simulink model "is95fwdchcodec"  (Simulink 4.00)
settings: Solver=VariableStepDiscrete  SolverMode=SingleTasking  StartTime=0.0  StopTime=20.0  RelTol=1e-3  AbsTol=1e-6
undefined symbols (not defined in the file or in its folder): slcm
libraries: cdmalib x8, dspsrcs2 x3, dspmtrx2 x2, commsink x2, commchan x1
settings Model: Creator=rkumar  LastModifiedBy=akansal  SaveTime=off  SaveOutput=off  LimitDataPoints=off  ExtModeTrigMode=oneshot  ExtModeArmWhenConnect=off  BlockReductionOpt=off

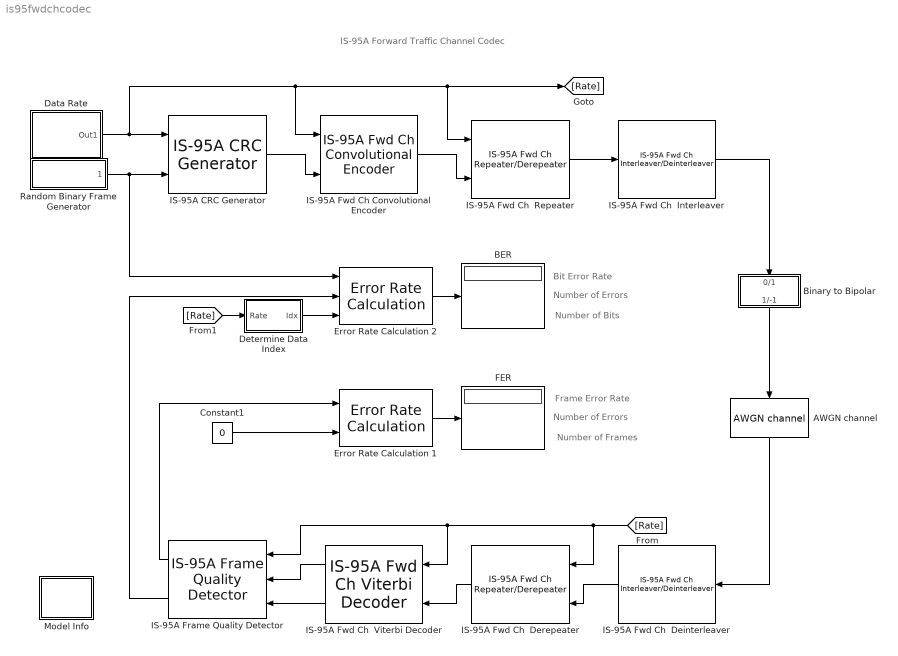
== system is95fwdchcodec ==
  note: IS-95A Forward Traffic Channel Codec
  note: Frame Error Rate
  note: Number of Errors
  note: Number of Frames
  note: Bit Error Rate
  note: Number of Errors
  note: Number of Bits
  AWGN channel : commchan/AWGN channel  Orientation=down  seed=11243  noiseMode="Signal to noise ratio  (SNR)"  EsNodB=-1  SNRdB=2  Ps=1  Tsym=1/(50*384)  variance=1  FrameBased=on  nChans=1
  BER : Display
      settings: Format=short
  Binary to Bipolar : Subsystem  Orientation=down
      settings: RTWFcnNameOpts=Auto  RTWFileNameOpts=Auto
      mask Type: Binary to Bipolar Transformation
      mask Description: Binary to Bipolar Transformation.
      mask Display: disp('0/1->1/-1')
  Constant1 : Constant  Value=0
  Data Rate : Subsystem  mask{rate=Full}
      mask prompts: rate "Data Rate"
      settings: RTWFcnNameOpts=Auto  RTWFileNameOpts=Auto
      mask StyleString: popup(Full|Half|Quarter|One-Eighth)
      mask Display: disp('Base Station \nTransmitter\nData Rate')
  Determine Data Index : Subsystem  mask(Determine Data Index){rateSet=Rate Set I}
      mask prompts: rateSet "Rate set:"
      mask help: Deterime index of valid data in the frame based upon rate set and rate input.
      mask init:
      | if(rateSet==1)
      | % --- Rate Set 1
      |    R1F = buffer(1:172,268);
      |    R1H = buffer(1:80,268);
      |    R1Q = buffer(1:40,268);
      |    R1E = buffer(1:16,268);
      |    idxMat = [R1F R1H R1Q R1E];
      | else
      |    % --- Rate Set 2
      |    R2F = [1:268]';
      |    R2H = buffer(1:126,268);
      |    R2Q = buffer(1:56,268);
      |    R2E = buffer(1:22,268);
      |    idxMat = [R2F R2H R2Q R2E];
      | end;
      settings: RTWFcnNameOpts=Auto  RTWFileNameOpts=Auto
      mask StyleString: popup(Rate Set I|Rate Set II)
  Error Rate Calculation 1 : commsink/Error Rate Calculation  N=0  st_delay=4  cp_mode=Entire frame  subframe=[]  PMode=Port  WsName=ErrorVec  RsMode2=off
  Error Rate Calculation 2 : commsink/Error Rate Calculation  N=0  st_delay=4*268  cp_mode=Select samples from port  subframe=[]  PMode=Port  WsName=ErrorVec  RsMode2=off
  FER : Display
      settings: Format=short
  IS-95A CRC Generator : cdmalib/IS-95A Common/IS-95A CRC Generator  rate_set=Rate Set I  ch_type=Traffic
  IS-95A Frame Quality Detector : cdmalib/IS-95A Common/IS-95A Frame Quality  Detector  Orientation=left  rateSet=Rate Set I  chType=Traffic  rate2_metric=0.9*1.5  rate3_metric=0.85*1.5
  IS-95A Fwd Ch Convolutional Encoder : cdmalib/IS-95A Base Station Transmitter/IS-95A Fwd Ch Convolutional Encoder  rate_set=Rate Set I  ch_type=Traffic  enc_state=[]
  IS-95A Fwd Ch  Deinterleaver : cdmalib/IS-95A Base Station Transmitter/IS-95A Fwd Ch Interleaver//Deinterleaver  Orientation=left  ch_type=Traffic  int_select=Deinterleaver
  IS-95A Fwd Ch  Derepeater : cdmalib/IS-95A Base Station Transmitter/IS-95A Fwd Ch Repeater//Derepeater  Orientation=left  rate_set=Rate Set I  ch_type=Traffic  rep_select=Derepeater
  IS-95A Fwd Ch  Interleaver : cdmalib/IS-95A Base Station Transmitter/IS-95A Fwd Ch Interleaver//Deinterleaver  ch_type=Traffic  int_select=Interleaver
  IS-95A Fwd Ch  Repeater : cdmalib/IS-95A Base Station Transmitter/IS-95A Fwd Ch Repeater//Derepeater  rate_set=Rate Set I  ch_type=Traffic  rep_select=Repeater
  IS-95A Fwd Ch  Viterbi Decoder : cdmalib/IS-95A Mobile Station Receiver/IS-95A Fwd Ch Viterbi Decoder  Orientation=left  rateSet=Rate Set I  chType=Traffic  traceBackLenRatio=1  decodeLenRatio=1
  Model Info : Subsystem  LoadFcn=slcm LoadBlock;  InitFcn=slcm('UpdateAllCMBlocksInThisModelInit')  mask(CMBlock){InitialSaveTempField=, InitialBlockCM=none, BlockCM=none, Frame=on, SaveTempField=, DisplayStringWithTags=Info, MaskDisplayString=Info, HorizontalTextAlignment=Center, LeftAlignmentValue=0.5, SourceBlockDiagram=is95fwdchcodec, TagMaxNumber=20, CMTag1=, CMTag2=, CMTag3=, CMTag4=, CMTag5=, CMTag6=, CMTag7=, CMTag8=, CMTag9=, CMTag10=, CMTag11=, CMTag12=, CMTag13=, CMTag14=, CMTag15=, CMTag16=, CMTag17=, CMTag18=, CMTag19=, CMTag20=}
      mask help: This block allows revision control information to be displayed within the model.
      settings: CopyFcn=slcm CopyBlock;  DeleteFcn=slcm Cancel;  PostSaveFcn=slcm('UpdateAllCMBlocksInThisModel')  NameChangeFcn=slcm Rename;  OpenFcn=cdmademohelp;  RTWFcnNameOpts=Auto  RTWFileNameOpts=Auto
      mask Display: text(str2num(LeftAlignmentValue), 0.5, MaskDisplayString, 'HorizontalAlignment', HorizontalTextAlignment)
  Random Binary Frame Generator : Subsystem  mask(Random Binary Frame Generator){seed=119940, Ts=1/(50*268), N=268}
      mask prompts: seed "Initial seed:"; Ts "Sample time (sec):"; N "Output frame size:"
      mask help:
      | Generate a random frame of binary integers. The output frame period is
      | (Sample time) * (Output frame size).
      settings: RTWFcnNameOpts=Auto  RTWFileNameOpts=Auto
      mask Display: plot(0,0,100,100,[95,90,90,80,80,60,60,30,30,20,20,10,10,5],[25,25,75,75,25,25,75,75,25,25,75,75,25,25]);
  wires:
  IS-95A Fwd Ch  Repeater/1 -> IS-95A Fwd Ch  Interleaver/1
  Data Rate/1(Out1) -> IS-95A Fwd Ch Convolutional Encoder/1, IS-95A Fwd Ch  Repeater/1, [Rate], IS-95A CRC Generator/1
  IS-95A Fwd Ch  Interleaver/1 -> Binary to Bipolar/1(0/1)
  Binary to Bipolar/1(1/-1) -> AWGN channel/1
  IS-95A Fwd Ch Convolutional Encoder/1 -> IS-95A Fwd Ch  Repeater/2
  IS-95A CRC Generator/1 -> IS-95A Fwd Ch Convolutional Encoder/2
  AWGN channel/1 -> IS-95A Fwd Ch  Deinterleaver/1
  IS-95A Fwd Ch  Deinterleaver/1 -> IS-95A Fwd Ch  Derepeater/2
  IS-95A Fwd Ch  Derepeater/1 -> IS-95A Fwd Ch  Viterbi Decoder/2
  IS-95A Fwd Ch  Viterbi Decoder/1 -> IS-95A Frame Quality Detector/2
  IS-95A Fwd Ch  Viterbi Decoder/2 -> IS-95A Frame Quality Detector/3
  [Rate] -> IS-95A Fwd Ch  Derepeater/1, IS-95A Fwd Ch  Viterbi Decoder/1, IS-95A Frame Quality Detector/1
  Error Rate Calculation 2/1 -> BER/1
  [Rate] -> Determine Data Index/1(Rate)
  Determine Data Index/1(Idx) -> Error Rate Calculation 2/3
  Error Rate Calculation 1/1 -> FER/1
  Constant1/1 -> Error Rate Calculation 1/2
  IS-95A Frame Quality Detector/2 -> Error Rate Calculation 2/2
  IS-95A Frame Quality Detector/1 -> Error Rate Calculation 1/1
  Random Binary Frame Generator/1(" ") -> IS-95A CRC Generator/2, Error Rate Calculation 2/1

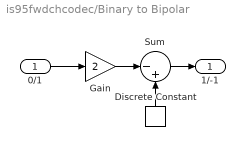
== system is95fwdchcodec/Binary to Bipolar ==
  0/1 : Inport  Port=1
  Discrete Constant : dspsrcs2/Discrete Constant  Orientation=up  Value=1  Ts=1/50
  Gain : Gain  Gain=2  Multiplication=Element-wise(K.*u)  SaturateOnIntegerOverflow=on
  Sum : Sum  Inputs=|-+  SaturateOnIntegerOverflow=on
  1/-1 : Outport  Port=1  InitialOutput=0
  wires:
  Sum/1 -> 1/-1/1
  Gain/1 -> Sum/1
  0/1/1 -> Gain/1
  Discrete Constant/1 -> Sum/2

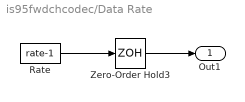
== system is95fwdchcodec/Data Rate ==
  Rate : Constant  Value=rate-1
  Zero-Order Hold3 : ZeroOrderHold  SampleTime=1/50
  Out1 : Outport  Port=1  InitialOutput=0
  wires:
  Zero-Order Hold3/1 -> Out1/1
  Rate/1 -> Zero-Order Hold3/1

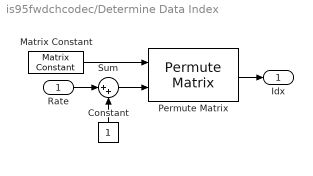
== system is95fwdchcodec/Determine Data Index ==
  Rate : Inport  Port=1
  Constant : Constant  Orientation=up  Value=1
  Matrix Constant : dspmtrx2/Matrix Constant  M=idxMat
  Permute Matrix : dspmtrx2/Permute Matrix  mode=Columns  errmode=Clip Index  cols=4
  Sum : Sum  Inputs=|++  SaturateOnIntegerOverflow=on
  Idx : Outport  Port=1
  wires:
  Constant/1 -> Sum/2
  Matrix Constant/1 -> Permute Matrix/1
  Permute Matrix/1 -> Idx/1
  Sum/1 -> Permute Matrix/2
  Rate/1 -> Sum/1

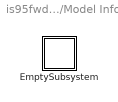
== system is95fwdchcodec/Model Info ==
  EmptySubsystem : Subsystem
      settings: RTWFcnNameOpts=Auto  RTWFileNameOpts=Auto

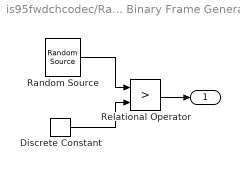
== system is95fwdchcodec/Random Binary Frame Generator ==
  Discrete Constant : dspsrcs2/Discrete Constant  Value=0.5  Ts=Ts*N
  Random Source : dspsrcs2/Random Source  SrcType=Uniform  Min=0  Max=1  Mean=0  Var=1  Seed=seed  SampMode=Discrete  Inherit=off  SampTime=Ts  SampFrame=N  OutComplex=Real
  Relational Operator : RelationalOperator  Operator=>
  " " : Outport  Port=1
  wires:
  Random Source/1 -> Relational Operator/1
  Discrete Constant/1 -> Relational Operator/2
  Relational Operator/1 -> " "/1

== system is95fwdchcodec/Model Info/EmptySubsystem ==
